simulink model "RobotModel5"  (R2025b)
settings: Solver=VariableStepAuto  StartTime=0.0  StopTime=80  RelTol=0.01  AbsTol=0.01  EnableMultiTasking=on
values from neighbouring files (symbols this model uses):
  waypoints = [R*cos(theta)+5, R*sin(theta)]    [init_waypoints.m]
undefined symbols (not defined in the file or in its folder): X, Y, Z
libraries: sm_lib x70, nesl_utility x45, slpidlib x2, robotalgslib x1, sharedtransform x1
(part 4 of 4)

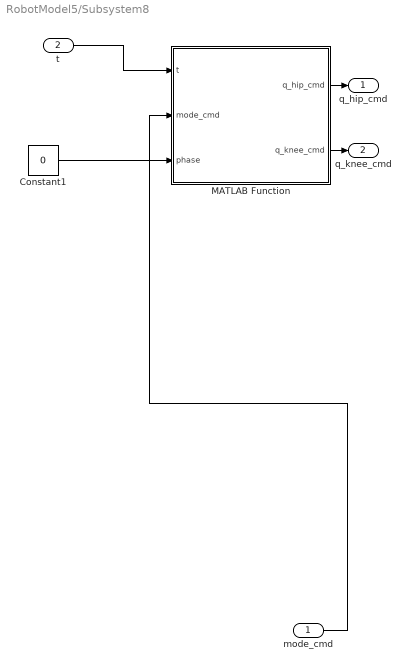
== system RobotModel5/Subsystem8 ==
  mode_cmd : Inport
  t : Inport  Port=2
  Constant1 : Constant  Value=0
  MATLAB Function : MATLAB Function  TreatAsAtomicUnit=on
  q_hip_cmd : Outport
  q_knee_cmd : Outport  Port=2
  wires:
  Constant1/1 -> MATLAB Function/3(phase)
  mode_cmd/1 -> MATLAB Function/2(mode_cmd)
  MATLAB Function/1(q_hip_cmd) -> q_hip_cmd/1
  MATLAB Function/2(q_knee_cmd) -> q_knee_cmd/1
  t/1 -> MATLAB Function/1(t)

== system RobotModel5/Subsystem9 ==
  mode_cmd : Inport
  t : Inport  Port=2
  Constant1 : Constant  Value=0.25
  MATLAB Function : MATLAB Function  TreatAsAtomicUnit=on
  q_hip_cmd : Outport
  q_knee_cmd : Outport  Port=2
  wires:
  t/1 -> MATLAB Function/1(t)
  Constant1/1 -> MATLAB Function/3(phase)
  mode_cmd/1 -> MATLAB Function/2(mode_cmd)
  MATLAB Function/1(q_hip_cmd) -> q_hip_cmd/1
  MATLAB Function/2(q_knee_cmd) -> q_knee_cmd/1

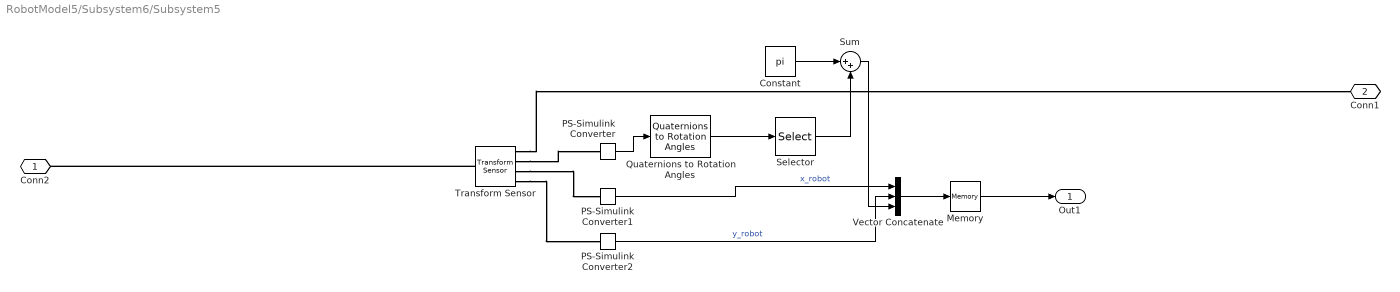
== system RobotModel5/Subsystem6/Subsystem5 ==
  Constant : Constant  Value=pi
  Memory : Memory
  PS-Simulink Converter : nesl_utility/PS-Simulink Converter  PhysicalDomain=network_engine_domain  SubClassName=ps_output  LeftPortType=input  RightPortType=output  PseudoPeriodic=off  Frequencies=[]  VectorFormat=inherit  Unit=inherit  AffineConversion=off
  PS-Simulink Converter1 : nesl_utility/PS-Simulink Converter  PhysicalDomain=network_engine_domain  SubClassName=ps_output  LeftPortType=input  RightPortType=output  PseudoPeriodic=off  Frequencies=[]  VectorFormat=inherit  Unit=inherit  AffineConversion=off
  PS-Simulink Converter2 : nesl_utility/PS-Simulink Converter  PhysicalDomain=network_engine_domain  SubClassName=ps_output  LeftPortType=input  RightPortType=output  PseudoPeriodic=off  Frequencies=[]  VectorFormat=inherit  Unit=inherit  AffineConversion=off
  Quaternions to Rotation Angles : sharedtransform/Quaternions to Rotation Angles  rotationOrder=ZYX  aMode=aMode
  Selector : Selector  InputPortWidth=3  IndexOptions=Index vector (dialog)  Indices=[1]  OutputSizes=1
  Sum : Sum  Inputs=|++
  Transform Sensor : sm_lib/Frames and Transforms/Transform Sensor  MeasurementFrame=World  RotationSequence=XYX  SenseAngle=off  SenseAxis=off  SenseQ=on  SenseR=off  SenseRotationSequence=off  SenseOmegaX=off  SenseOmegaY=off  SenseOmegaZ=off  SenseOmega=off  SenseQDot=off  SenseRDot=off  SenseRotationSequenceDot=off  SenseAlphaX=off  SenseAlphaY=off  SenseAlphaZ=off  SenseAlpha=off  SenseQDDot=off  SenseRDDot=off  SenseX=on  SenseY=on  SenseZ=off  SenseXYZ=off  SenseRad=off  SenseAzim=off  SenseDist=off  SenseInc=off  SenseXDot=off  SenseYDot=off  SenseZDot=off  SenseXYZDot=off  SenseRadDot=off  SenseAzimDot=off  SenseDistDot=off  SenseIncDot=off  SenseXDDot=off  SenseYDDot=off  SenseZDDot=off  SenseXYZDDot=off  SenseRadDDot=off  SenseAzimDDot=off  SenseDistDDot=off  SenseIncDDot=off
  Vector Concatenate : Concatenate  NumInputs=3
  Conn2 : PMIOPort  Side=Left
  Conn1 : PMIOPort  Port=2  Side=Right
  Out1 : Outport
  wires:
  Quaternions to Rotation Angles/1 -> Selector/1
  PS-Simulink Converter/1 -> Quaternions to Rotation Angles/1
  Vector Concatenate/1 -> Memory/1
  Memory/1 -> Out1/1
  PS-Simulink Converter1/1 -> Vector Concatenate/1  "x_robot"
  PS-Simulink Converter2/1 -> Vector Concatenate/2  "y_robot"
  Selector/1 -> Sum/2
  Constant/1 -> Sum/1
  Sum/1 -> Vector Concatenate/3
  connections:
  Transform Sensor/LConn1 -- Conn2/RConn1
  Transform Sensor/RConn4 -- PS-Simulink Converter2/LConn1
  Transform Sensor/RConn2 -- PS-Simulink Converter/LConn1
  Transform Sensor/RConn3 -- PS-Simulink Converter1/LConn1
  Transform Sensor/RConn1 -- Conn1/RConn1

== matlab function RobotModel5/Subsystem4/MATLAB Function1 ==
  data: mode_cmd input; alpha input; tau output; q input; dq input; q_cmd input; is_locked output; q_ref output
function [tau, is_locked, q_ref] = LockJointPD(mode_cmd, alpha, q, dq, q_cmd)
%#codegen
% mode_cmd: 0=Walk (track q_cmd), 1=Wheeled (lock current angle)
% alpha   : [0,1] smoothing factor (TransferFcn output), 0=fully walking, 1=fully locked
% q,dq    : joint angle/angular velocity
% q_cmd   : walk/stand target angle (radians)
Kp = 1200.0;   % Starting value, tune per joint
Kd =   20.0;
tau_lim = 300.0;
m = uint8(mode_cmd ~= 0);     % Standardize to uint8(0/1)
a = double(alpha);
persistent q_hold last_mode
if isempty(q_hold),    q_hold    = q;        end   % double
if isempty(last_mode), last_mode = uint8(0); end   % uint8
% Rising edge: 0->1, latch current angle
if (last_mode == uint8(0)) && (m ~= uint8(0))
    q_hold = q;
end
last_mode = m;
% Reference angle: interpolate between "hold angle" and "target angle"
q_ref  = a*q_hold + (1-a)*q_cmd;
dq_ref = 0.0;
% PD
tau = Kp*(q_ref - q) + Kd*(dq_ref - dq);
% Saturation
tau = max(min(tau, tau_lim), -tau_lim);
% Debug flag: is leg lock dominant
is_locked = (a > 0.5);     % Can also output m==1
end

== matlab function RobotModel5/Subsystem6/MATLAB Function1 ==
  data: v input; wL_cmd output; w input; T input; r input; wR_cmd output
function [wL_cmd, wR_cmd] = wheelSpeedCmd(v, w, T, r)
% v: 线速度 [m/s]
% w: 航向角速度 [rad/s]
% T: 后轮距 [m]
% r: 车轮半径 [m]

vL = v - 0.5*T*w;
vR = v + 0.5*T*w;

wL_cmd = vL / r;
wR_cmd = vR / r;
end

== matlab function RobotModel5/Subsystem6/MATLAB Function ==
  data: v input; delta output; w input; L input; v output
function [delta, v] = Diff2Ackermann(v, w, L)
% input: 
%   v - Linear velocity (m/s)
%   w - Angular velocity (rad/s)
%   L -  (m)
%
% output:
%   delta - front wheel rotation angel (rad)
%   v     -  velocity(m/s)
if abs(v) < 1e-3
    delta = 0;
else
    delta = atan(L * w / v);   % pure pursuit function
end

== matlab function RobotModel5/Subsystem8/MATLAB Function ==
  data: t input; q_hip_cmd output; mode_cmd input; phase input; q_knee_cmd output
function [q_hip_cmd, q_knee_cmd] = StairLegTraj(t, mode_cmd, phase)
%#codegen
% ======== Tunable Parameters ========
T = 3.0;     % Total duration of one step, larger means slower
% Time ratio for the four phases: [Stand, Lift, Swing Over, Place]
s_stand = 0.30;
s_lift  = 0.65;
s_over  = 0.90;
% Remaining 0.90~1.00 is for placement
% --- Key Poses ---
hip_stand  = -0.2;
knee_stand =  0.3;
hip_lift   = -0.8;   % Leg lift: hip more negative, knee turns negative to bend
knee_lift  = -0.6;
hip_over   =  0.15;  % Forward swing over
knee_over  =  0.3;
hip_place  =  0.05;  % Foot placement pose
knee_place =  0.3;
% ======== Wheeled Mode: Maintain Stand ========
if mode_cmd ~= 0
    q_hip_cmd  = 0;
    q_knee_cmd = 0;
    return;
end
% ======== Normalized time s ∈ [0,1) ========
tau = mod(t + phase*T, T);
s   = tau / T;
% Helper: smooth interpolation 0→1 (S-curve, avoid burst)
smooth = @(u) (u.^2 .* (3 - 2*u));   % 3u^2 - 2u^3
if s < s_stand
    % Phase 1: Stand
    q_hip_cmd  = hip_stand;
    q_knee_cmd = knee_stand;
elseif s < s_lift
    % Phase 2: Slowly lift leg (longer duration)
    u = (s - s_stand) / (s_lift - s_stand);   % 0→1
    u = smooth(u);
    q_hip_cmd  = (1-u)*hip_stand  + u*hip_lift;
    q_knee_cmd = (1-u)*knee_stand + u*knee_lift;
elseif s < s_over
    % Phase 3: From lift high to swing over
    u = (s - s_lift) / (s_over - s_lift);
    u = smooth(u);
    q_hip_cmd  = (1-u)*hip_lift  + u*hip_over;
    q_knee_cmd = (1-u)*knee_lift + u*knee_over;
else
    % Phase 4: From swing over to foot placement (also extended + smoothed to prevent harsh landing)
    u = (s - s_over) / (1 - s_over);
    u = smooth(u);
    q_hip_cmd  = (1-u)*hip_over  + u*hip_place;
    q_knee_cmd = (1-u)*knee_over + u*knee_place;
end
end

== matlab function RobotModel5/Subsystem9/MATLAB Function ==
  data: t input; q_hip_cmd output; mode_cmd input; phase input; q_knee_cmd output
function [q_hip_cmd, q_knee_cmd] = StairLegTraj(t, mode_cmd, phase)
%#codegen
% ======== Tunable Parameters ========
T = 3.0;     % Total duration of one step, larger means slower
% Time ratio for the four phases: [Stand, Lift, Swing Over, Place]
s_stand = 0.30;
s_lift  = 0.65;
s_over  = 0.90;
% Remaining 0.90~1.00 is for placement
% --- Key Poses ---
hip_stand  = -0.2;
knee_stand =  0.3;
hip_lift   = -0.8;   % Leg lift: hip more negative, knee turns negative to bend
knee_lift  = -0.6;
hip_over   =  0.15;  % Forward swing over
knee_over  =  0.3;
hip_place  =  0.05;  % Foot placement pose
knee_place =  0.3;
% ======== Wheeled Mode: Maintain Stand ========
if mode_cmd ~= 0
    q_hip_cmd  = 0;
    q_knee_cmd = 0;
    return;
end
% ======== Normalized time s ∈ [0,1) ========
tau = mod(t + phase*T, T);
s   = tau / T;
% Helper: smooth interpolation 0→1 (S-curve, avoid burst)
smooth = @(u) (u.^2 .* (3 - 2*u));   % 3u^2 - 2u^3
if s < s_stand
    % Phase 1: Stand
    q_hip_cmd  = hip_stand;
    q_knee_cmd = knee_stand;
elseif s < s_lift
    % Phase 2: Slowly lift leg (longer duration)
    u = (s - s_stand) / (s_lift - s_stand);   % 0→1
    u = smooth(u);
    q_hip_cmd  = (1-u)*hip_stand  + u*hip_lift;
    q_knee_cmd = (1-u)*knee_stand + u*knee_lift;
elseif s < s_over
    % Phase 3: From lift high to swing over
    u = (s - s_lift) / (s_over - s_lift);
    u = smooth(u);
    q_hip_cmd  = (1-u)*hip_lift  + u*hip_over;
    q_knee_cmd = (1-u)*knee_lift + u*knee_over;
else
    % Phase 4: From swing over to foot placement (also extended + smoothed to prevent harsh landing)
    u = (s - s_over) / (1 - s_over);
    u = smooth(u);
    q_hip_cmd  = (1-u)*hip_over  + u*hip_place;
    q_knee_cmd = (1-u)*knee_over + u*knee_place;
end
end

== matlab function RobotModel5/Subsystem10/MATLAB Function ==
  data: t input; q_hip_cmd output; mode_cmd input; phase input; q_knee_cmd output
function [q_hip_cmd, q_knee_cmd] = StairLegTraj(t, mode_cmd, phase)
%#codegen
% ======== Tunable Parameters ========
T = 3.0;     % Total duration of one step, larger means slower
% Time ratio for the four phases: [Stand, Lift, Swing Over, Place]
s_stand = 0.30;
s_lift  = 0.65;
s_over  = 0.90;
% Remaining 0.90~1.00 is for placement
% --- Key Poses ---
hip_stand  = -0.2;
knee_stand =  0.3;
hip_lift   = -0.8;   % Leg lift: hip more negative, knee turns negative to bend
knee_lift  = -0.6;
hip_over   =  0.15;  % Forward swing over
knee_over  =  0.3;
hip_place  =  0.05;  % Foot placement pose
knee_place =  0.3;
% ======== Wheeled Mode: Maintain Stand ========
if mode_cmd ~= 0
    q_hip_cmd  = 0;
    q_knee_cmd = 0;
    return;
end
% ======== Normalized time s ∈ [0,1) ========
tau = mod(t + phase*T, T);
s   = tau / T;
% Helper: smooth interpolation 0→1 (S-curve, avoid burst)
smooth = @(u) (u.^2 .* (3 - 2*u));   % 3u^2 - 2u^3
if s < s_stand
    % Phase 1: Stand
    q_hip_cmd  = hip_stand;
    q_knee_cmd = knee_stand;
elseif s < s_lift
    % Phase 2: Slowly lift leg (longer duration)
    u = (s - s_stand) / (s_lift - s_stand);   % 0→1
    u = smooth(u);
    q_hip_cmd  = (1-u)*hip_stand  + u*hip_lift;
    q_knee_cmd = (1-u)*knee_stand + u*knee_lift;
elseif s < s_over
    % Phase 3: From lift high to swing over
    u = (s - s_lift) / (s_over - s_lift);
    u = smooth(u);
    q_hip_cmd  = (1-u)*hip_lift  + u*hip_over;
    q_knee_cmd = (1-u)*knee_lift + u*knee_over;
else
    % Phase 4: From swing over to foot placement (also extended + smoothed to prevent harsh landing)
    u = (s - s_over) / (1 - s_over);
    u = smooth(u);
    q_hip_cmd  = (1-u)*hip_over  + u*hip_place;
    q_knee_cmd = (1-u)*knee_over + u*knee_place;
end
end

== matlab function RobotModel5/Subsystem1/MATLAB Function1 ==
  data: mode_cmd input; alpha input; tau output; q input; dq input; q_cmd input; is_locked output; q_ref output
function [tau, is_locked, q_ref] = LockJointPD(mode_cmd, alpha, q, dq, q_cmd)
%#codegen
% mode_cmd: 0=Walk (track q_cmd), 1=Wheeled (lock current angle)
% alpha   : [0,1] smoothing factor (TransferFcn output), 0=fully walking, 1=fully locked
% q,dq    : joint angle/angular velocity
% q_cmd   : walk/stand target angle (radians)
Kp = 1200.0;   % Starting value, tune per joint
Kd =   20.0;
tau_lim = 300.0;
m = uint8(mode_cmd ~= 0);     % Standardize to uint8(0/1)
a = double(alpha);
persistent q_hold last_mode
if isempty(q_hold),    q_hold    = q;        end   % double
if isempty(last_mode), last_mode = uint8(0); end   % uint8
% Rising edge: 0->1, latch current angle
if (last_mode == uint8(0)) && (m ~= uint8(0))
    q_hold = q;
end
last_mode = m;
% Reference angle: interpolate between "hold angle" and "target angle"
q_ref  = a*q_hold + (1-a)*q_cmd;
dq_ref = 0.0;
% PD
tau = Kp*(q_ref - q) + Kd*(dq_ref - dq);
% Saturation
tau = max(min(tau, tau_lim), -tau_lim);
% Debug flag: is leg lock dominant
is_locked = (a > 0.5);     % Can also output m==1
end

== matlab function RobotModel5/Subsystem11/MATLAB Function ==
  data: t input; q_hip_cmd output; mode_cmd input; phase input; q_knee_cmd output
function [q_hip_cmd, q_knee_cmd] = StairLegTraj(t, mode_cmd, phase)
%#codegen
% ======== Tunable Parameters ========
T = 3.0;     % Total duration of one step, larger means slower
% Time ratio for the four phases: [Stand, Lift, Swing Over, Place]
s_stand = 0.30;
s_lift  = 0.65;
s_over  = 0.90;
% Remaining 0.90~1.00 is for placement
% --- Key Poses ---
hip_stand  = -0.2;
knee_stand =  0.3;
hip_lift   = -0.8;   % Leg lift: hip more negative, knee turns negative to bend
knee_lift  = -0.6;
hip_over   =  0.15;  % Forward swing over
knee_over  =  0.3;
hip_place  =  0.05;  % Foot placement pose
knee_place =  0.3;
% ======== Wheeled Mode: Maintain Stand ========
if mode_cmd ~= 0
    q_hip_cmd  = 0;
    q_knee_cmd = 0;
    return;
end
% ======== Normalized time s ∈ [0,1) ========
tau = mod(t + phase*T, T);
s   = tau / T;
% Helper: smooth interpolation 0→1 (S-curve, avoid burst)
smooth = @(u) (u.^2 .* (3 - 2*u));   % 3u^2 - 2u^3
if s < s_stand
    % Phase 1: Stand
    q_hip_cmd  = hip_stand;
    q_knee_cmd = knee_stand;
elseif s < s_lift
    % Phase 2: Slowly lift leg (longer duration)
    u = (s - s_stand) / (s_lift - s_stand);   % 0→1
    u = smooth(u);
    q_hip_cmd  = (1-u)*hip_stand  + u*hip_lift;
    q_knee_cmd = (1-u)*knee_stand + u*knee_lift;
elseif s < s_over
    % Phase 3: From lift high to swing over
    u = (s - s_lift) / (s_over - s_lift);
    u = smooth(u);
    q_hip_cmd  = (1-u)*hip_lift  + u*hip_over;
    q_knee_cmd = (1-u)*knee_lift + u*knee_over;
else
    % Phase 4: From swing over to foot placement (also extended + smoothed to prevent harsh landing)
    u = (s - s_over) / (1 - s_over);
    u = smooth(u);
    q_hip_cmd  = (1-u)*hip_over  + u*hip_place;
    q_knee_cmd = (1-u)*knee_over + u*knee_place;
end
end

== matlab function RobotModel5/Subsystem1/MATLAB Function2 ==
  settings: updateMethod=DISCRETE
  data: mode_cmd input; tau output; q input; dq input
function tau = WheelLockPD(mode_cmd, q, dq)
%#codegen
% mode_cmd: 0=Walk (lock wheel), 1=Wheeled (don't lock wheel)
% q, dq measurements from the wheel axle Revolute Joint
% Braking PD parameters (tunable)
Kp = 500.0;     % Braking stiffness, smaller to avoid being too rigid
Kd =  20.0;     % Damping
tau_lim = 150.0;  % Maximum braking torque for the wheel
% Lock only in walk mode
lock = (mode_cmd == 0);
persistent q_hold last_lock
if isempty(q_hold),    q_hold    = q;     end
if isempty(last_lock), last_lock = false; end
% The moment it switches from "unlocked" to "locked", remember the current angle
if (~last_lock) && lock
    q_hold = q;
end
last_lock = lock;
if lock
    % Lock wheel: treat q_hold as the target angle
    q_ref  = q_hold;
    dq_ref = 0.0;
    tau = Kp*(q_ref - q) + Kd*(dq_ref - dq);
else
    % Wheeled mode: do not apply brake
    tau = 0.0;
end
% Torque saturation
if tau >  tau_lim, tau =  tau_lim; end
if tau < -tau_lim, tau = -tau_lim; end
end

== matlab function RobotModel5/Subsystem2/MATLAB Function2 ==
  settings: updateMethod=DISCRETE
  data: mode_cmd input; tau output; q input; dq input
function tau = WheelLockPD(mode_cmd, q, dq)
%#codegen
% mode_cmd: 0=Walk (lock wheel), 1=Wheeled (don't lock wheel)
% q, dq measurements from the wheel axle Revolute Joint
% Braking PD parameters (tunable)
Kp = 500.0;     % Braking stiffness, smaller to avoid being too rigid
Kd =  20.0;     % Damping
tau_lim = 150.0;  % Maximum braking torque for the wheel
% Lock only in walk mode
lock = (mode_cmd == 0);
persistent q_hold last_lock
if isempty(q_hold),    q_hold    = q;     end
if isempty(last_lock), last_lock = false; end
% The moment it switches from "unlocked" to "locked", remember the current angle
if (~last_lock) && lock
    q_hold = q;
end
last_lock = lock;
if lock
    % Lock wheel: treat q_hold as the target angle
    q_ref  = q_hold;
    dq_ref = 0.0;
    tau = Kp*(q_ref - q) + Kd*(dq_ref - dq);
else
    % Wheeled mode: do not apply brake
    tau = 0.0;
end
% Torque saturation
if tau >  tau_lim, tau =  tau_lim; end
if tau < -tau_lim, tau = -tau_lim; end
end

== matlab function RobotModel5/Subsystem4/MATLAB Function2 ==
  settings: updateMethod=DISCRETE
  data: mode_cmd input; tau output; q input; dq input
function tau = WheelLockPD(mode_cmd, q, dq)
%#codegen
% mode_cmd: 0=Walk (lock wheel), 1=Wheeled (don't lock wheel)
% q, dq measurements from the wheel axle Revolute Joint
% Braking PD parameters (tunable)
Kp = 500.0;     % Braking stiffness, smaller to avoid being too rigid
Kd =  20.0;     % Damping
tau_lim = 150.0;  % Maximum braking torque for the wheel
% Lock only in walk mode
lock = (mode_cmd == 0);
persistent q_hold last_lock
if isempty(q_hold),    q_hold    = q;     end
if isempty(last_lock), last_lock = false; end
% The moment it switches from "unlocked" to "locked", remember the current angle
if (~last_lock) && lock
    q_hold = q;
end
last_lock = lock;
if lock
    % Lock wheel: treat q_hold as the target angle
    q_ref  = q_hold;
    dq_ref = 0.0;
    tau = Kp*(q_ref - q) + Kd*(dq_ref - dq);
else
    % Wheeled mode: do not apply brake
    tau = 0.0;
end
% Torque saturation
if tau >  tau_lim, tau =  tau_lim; end
if tau < -tau_lim, tau = -tau_lim; end
end

== matlab function RobotModel5/Subsystem3/MATLAB Function2 ==
  settings: updateMethod=DISCRETE
  data: mode_cmd input; tau output; q input; dq input
function tau = WheelLockPD(mode_cmd, q, dq)
%#codegen
% mode_cmd: 0=Walk (lock wheel), 1=Wheeled (don't lock wheel)
% q, dq measurements from the wheel axle Revolute Joint
% Braking PD parameters (tunable)
Kp = 500.0;     % Braking stiffness, smaller to avoid being too rigid
Kd =  20.0;     % Damping
tau_lim = 150.0;  % Maximum braking torque for the wheel
% Lock only in walk mode
lock = (mode_cmd == 0);
persistent q_hold last_lock
if isempty(q_hold),    q_hold    = q;     end
if isempty(last_lock), last_lock = false; end
% The moment it switches from "unlocked" to "locked", remember the current angle
if (~last_lock) && lock
    q_hold = q;
end
last_lock = lock;
if lock
    % Lock wheel: treat q_hold as the target angle
    q_ref  = q_hold;
    dq_ref = 0.0;
    tau = Kp*(q_ref - q) + Kd*(dq_ref - dq);
else
    % Wheeled mode: do not apply brake
    tau = 0.0;
end
% Torque saturation
if tau >  tau_lim, tau =  tau_lim; end
if tau < -tau_lim, tau = -tau_lim; end
end

== matlab function RobotModel5/Subsystem1/MATLAB Function ==
  data: mode_cmd input; alpha input; tau output; q input; dq input; q_cmd input; is_locked output; q_ref output
function [tau, is_locked, q_ref] = LockJointPD(mode_cmd, alpha, q, dq, q_cmd)
%#codegen
% mode_cmd: 0=Walk(folloew q_cmd), 1=Wheel(lock the present angle )
% alpha   : [0,1] flatten faktor(TransferFcnoutput)，0=walk, 1=leg locked
% q,dq    : joint angle/angular velocity
% q_cmd   : walking/standing angle(rad)

Kp = 1200.0;   % start value
Kd =   20.0;
tau_lim = 300.0;

m = uint8(mode_cmd ~= 0);     % uint8(0/1)
a = double(alpha);

persistent q_hold last_mode
if isempty(q_hold),    q_hold    = q;        end   % double
if isempty(last_mode), last_mode = uint8(0); end   % uint8

% step: 0->1 
if (last_mode == uint8(0)) && (m ~= uint8(0))
    q_hold = q;
end
last_mode = m;

% reference angle
q_ref  = a*q_hold + (1-a)*q_cmd;
dq_ref = 0.0;

% PD
tau = Kp*(q_ref - q) + Kd*(dq_ref - dq);

% 
tau = max(min(tau, tau_lim), -tau_lim);

% 
is_locked = (a > 0.5);     % 
end

== matlab function RobotModel5/Subsystem2/MATLAB Function ==
  data: mode_cmd input; alpha input; tau output; q input; dq input; q_cmd input; is_locked output; q_ref output
function [tau, is_locked, q_ref] = LockJointPD(mode_cmd, alpha, q, dq, q_cmd)
%#codegen
% mode_cmd: 0=Walk (track q_cmd), 1=Wheeled (lock current angle)
% alpha   : [0,1] smoothing factor (TransferFcn output), 0=fully walking, 1=fully locked
% q,dq    : joint angle/angular velocity
% q_cmd   : walk/stand target angle (radians)
Kp = 1200.0;   % Starting value, tune per joint
Kd =   20.0;
tau_lim = 300.0;
m = uint8(mode_cmd ~= 0);     % Standardize to uint8(0/1)
a = double(alpha);
persistent q_hold last_mode
if isempty(q_hold),    q_hold    = q;        end   % double
if isempty(last_mode), last_mode = uint8(0); end   % uint8
% Rising edge: 0->1, latch current angle
if (last_mode == uint8(0)) && (m ~= uint8(0))
    q_hold = q;
end
last_mode = m;
% Reference angle: interpolate between "hold angle" and "target angle"
q_ref  = a*q_hold + (1-a)*q_cmd;
dq_ref = 0.0;
% PD
tau = Kp*(q_ref - q) + Kd*(dq_ref - dq);
% Saturation
tau = max(min(tau, tau_lim), -tau_lim);
% Debug flag: is leg lock dominant
is_locked = (a > 0.5);     % Can also output m==1
end

== matlab function RobotModel5/Subsystem2/MATLAB Function1 ==
  data: mode_cmd input; alpha input; tau output; q input; dq input; q_cmd input; is_locked output; q_ref output
function [tau, is_locked, q_ref] = LockJointPD(mode_cmd, alpha, q, dq, q_cmd)
%#codegen
% mode_cmd: 0=Walk (track q_cmd), 1=Wheeled (lock current angle)
% alpha   : [0,1] smoothing factor (TransferFcn output), 0=fully walking, 1=fully locked
% q,dq    : joint angle/angular velocity
% q_cmd   : walk/stand target angle (radians)
Kp = 1200.0;   % Starting value, tune per joint
Kd =   20.0;
tau_lim = 300.0;
m = uint8(mode_cmd ~= 0);     % Standardize to uint8(0/1)
a = double(alpha);
persistent q_hold last_mode
if isempty(q_hold),    q_hold    = q;        end   % double
if isempty(last_mode), last_mode = uint8(0); end   % uint8
% Rising edge: 0->1, latch current angle
if (last_mode == uint8(0)) && (m ~= uint8(0))
    q_hold = q;
end
last_mode = m;
% Reference angle: interpolate between "hold angle" and "target angle"
q_ref  = a*q_hold + (1-a)*q_cmd;
dq_ref = 0.0;
% PD
tau = Kp*(q_ref - q) + Kd*(dq_ref - dq);
% Saturation
tau = max(min(tau, tau_lim), -tau_lim);
% Debug flag: is leg lock dominant
is_locked = (a > 0.5);     % Can also output m==1
end

== matlab function RobotModel5/Subsystem3/MATLAB Function ==
  data: mode_cmd input; alpha input; tau output; q input; dq input; q_cmd input; is_locked output; q_ref output
function [tau, is_locked, q_ref] = LockJointPD(mode_cmd, alpha, q, dq, q_cmd)
%#codegen
% mode_cmd: 0=Walk (track q_cmd), 1=Wheeled (lock current angle)
% alpha   : [0,1] smoothing factor (TransferFcn output), 0=fully walking, 1=fully locked
% q,dq    : joint angle/angular velocity
% q_cmd   : walk/stand target angle (radians)
Kp = 1200.0;   % Starting value, tune per joint
Kd =   20.0;
tau_lim = 300.0;
m = uint8(mode_cmd ~= 0);     % Standardize to uint8(0/1)
a = double(alpha);
persistent q_hold last_mode
if isempty(q_hold),    q_hold    = q;        end   % double
if isempty(last_mode), last_mode = uint8(0); end   % uint8
% Rising edge: 0->1, latch current angle
if (last_mode == uint8(0)) && (m ~= uint8(0))
    q_hold = q;
end
last_mode = m;
% Reference angle: interpolate between "hold angle" and "target angle"
q_ref  = a*q_hold + (1-a)*q_cmd;
dq_ref = 0.0;
% PD
tau = Kp*(q_ref - q) + Kd*(dq_ref - dq);
% Saturation
tau = max(min(tau, tau_lim), -tau_lim);
% Debug flag: is leg lock dominant
is_locked = (a > 0.5);     % Can also output m==1
end

== matlab function RobotModel5/Subsystem3/MATLAB Function1 ==
  data: mode_cmd input; alpha input; tau output; q input; dq input; q_cmd input; is_locked output; q_ref output
function [tau, is_locked, q_ref] = LockJointPD(mode_cmd, alpha, q, dq, q_cmd)
%#codegen
% mode_cmd: 0=Walk (track q_cmd), 1=Wheeled (lock current angle)
% alpha   : [0,1] smoothing factor (TransferFcn output), 0=fully walking, 1=fully locked
% q,dq    : joint angle/angular velocity
% q_cmd   : walk/stand target angle (radians)
Kp = 1200.0;   % Starting value, tune per joint
Kd =   20.0;
tau_lim = 300.0;
m = uint8(mode_cmd ~= 0);     % Standardize to uint8(0/1)
a = double(alpha);
persistent q_hold last_mode
if isempty(q_hold),    q_hold    = q;        end   % double
if isempty(last_mode), last_mode = uint8(0); end   % uint8
% Rising edge: 0->1, latch current angle
if (last_mode == uint8(0)) && (m ~= uint8(0))
    q_hold = q;
end
last_mode = m;
% Reference angle: interpolate between "hold angle" and "target angle"
q_ref  = a*q_hold + (1-a)*q_cmd;
dq_ref = 0.0;
% PD
tau = Kp*(q_ref - q) + Kd*(dq_ref - dq);
% Saturation
tau = max(min(tau, tau_lim), -tau_lim);
% Debug flag: is leg lock dominant
is_locked = (a > 0.5);     % Can also output m==1
end

== matlab function RobotModel5/Subsystem4/MATLAB Function ==
  data: mode_cmd input; alpha input; tau output; q input; dq input; q_cmd input; is_locked output; q_ref output
function [tau, is_locked, q_ref] = LockJointPD(mode_cmd, alpha, q, dq, q_cmd)
%#codegen
% mode_cmd: 0=Walk (track q_cmd), 1=Wheeled (lock current angle)
% alpha   : [0,1] smoothing factor (TransferFcn output), 0=fully walking, 1=fully locked
% q,dq    : joint angle/angular velocity
% q_cmd   : walk/stand target angle (radians)
Kp = 1200.0;   % Starting value, tune per joint
Kd =   20.0;
tau_lim = 300.0;
m = uint8(mode_cmd ~= 0);     % Standardize to uint8(0/1)
a = double(alpha);
persistent q_hold last_mode
if isempty(q_hold),    q_hold    = q;        end   % double
if isempty(last_mode), last_mode = uint8(0); end   % uint8
% Rising edge: 0->1, latch current angle
if (last_mode == uint8(0)) && (m ~= uint8(0))
    q_hold = q;
end
last_mode = m;
% Reference angle: interpolate between "hold angle" and "target angle"
q_ref  = a*q_hold + (1-a)*q_cmd;
dq_ref = 0.0;
% PD
tau = Kp*(q_ref - q) + Kd*(dq_ref - dq);
% Saturation
tau = max(min(tau, tau_lim), -tau_lim);
% Debug flag: is leg lock dominant
is_locked = (a > 0.5);     % Can also output m==1
end
